simulink model "NEw"  (R2023a)
settings: Solver=FixedStepAuto  StartTime=0.0  StopTime=10  FixedStep=0.01  RelTol=1e-3  EnableMultiTasking=on
libraries: arduinolib x5, arduinosensorlib x1, SignalEditorBlockLib x1
settings Model: ExtModeTrigDuration=2  Creator=abdal  LastModifiedBy=abdal
settings OptimizationCC: EnhancedBackFolding=on  PassReuseOutputArgsAs=Individual arguments  ZeroExternalMemoryAtStartup=off  ZeroInternalMemoryAtStartup=off  MaxStackSize=64  OptimizeBlockOrder=speed  DifferentSizesBufferReuse=on  OptimizationCustomize=off  EfficientTunableParamExpr=on
settings DebuggingCC: ParameterPrecisionLossMsg=none  ParameterTunabilityLossMsg=error
settings HardwareCC: ProdBitPerInt=16  ProdBitPerPointer=16  ProdBitPerSizeT=16  ProdBitPerPtrDiffT=16  ProdLargestAtomicFloat=None  ProdWordSize=8  ProdLongLongMode=on  ProdHWDeviceType=Atmel->AVR
settings SFSimCC: MATLABDynamicMemAlloc=off
settings RTWCC: Description=Embedded Coder  SystemTargetFile=ert.tlc  HardwareBoard=Arduino Uno  TemplateMakefile=ert_default_tmf  Toolchain=Arduino AVR  BuildConfiguration=Faster Runs
settings CodeAppCC: ForceParamTrailComments=on  IgnoreCustomStorageClasses=off  OperatorAnnotations=on  SimulinkDataObjDesc=on  SFDataObjDesc=on  InsertBlockDesc=on
settings ERTTargetCC: SupportContinuousTime=on  SupportVariableSizeSignals=on  ExtModeTransport=3  ExtModeStaticAlloc=on  ExtModeAutomaticAllocSize=off  ExtModeStaticAllocSize=250  ExtModeMexFile=ext_xcp  ExtModeIntrfLevel=Level2 - Open

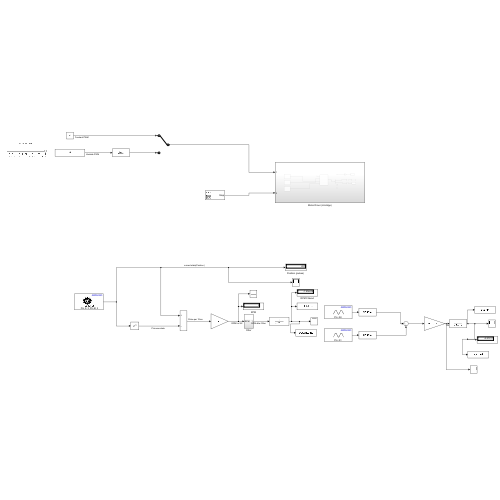
[thumbnail: Simulink's stored preview of the top-level diagram]
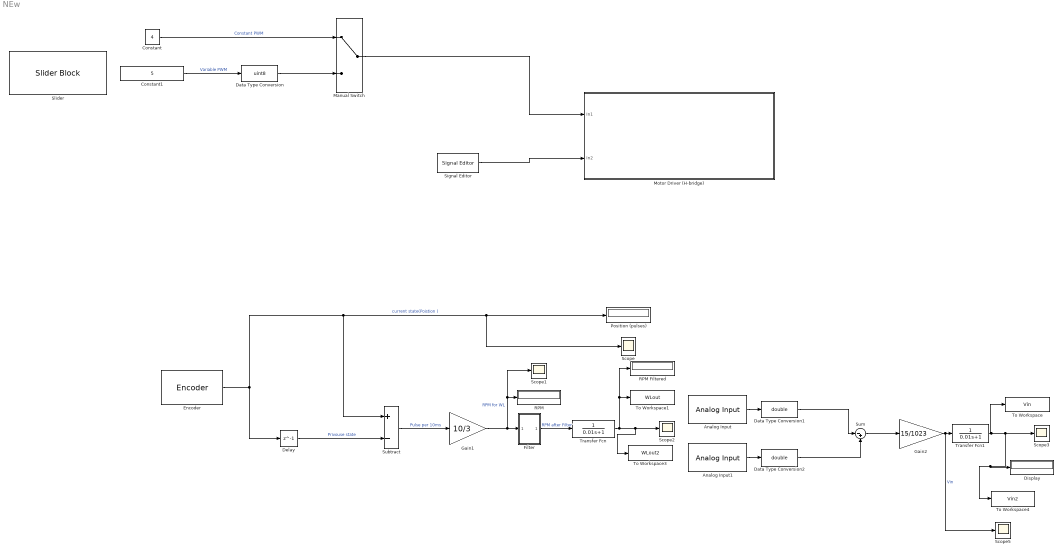
== system NEw ==
  Analog Input : arduinolib/Analog Input  pinNumber=0  ReadResultsOnly=off  ConversionTriggerSource=Software  ExternalTriggerType=uint32( 0 )  OutputDataType=uint16  EnableConversionCompleteNotify=off  EnableOuputStatus=off  SampleTime=-1  blockPlatform=arduino
  Analog Input1 : arduinolib/Analog Input  pinNumber=1  ReadResultsOnly=off  ConversionTriggerSource=Software  ExternalTriggerType=uint32( 0 )  OutputDataType=uint16  EnableConversionCompleteNotify=off  EnableOuputStatus=off  SampleTime=-1  blockPlatform=arduino
  Constant : Constant  Value=4
  Constant1 : Constant  Value=5
  Data Type Conversion : DataTypeConversion  OutMin=0  OutMax=255  OutDataTypeStr=uint8  RndMeth=Simplest  SaturateOnIntegerOverflow=off
  Data Type Conversion1 : DataTypeConversion  OutDataTypeStr=double  SaturateOnIntegerOverflow=off  RndMeth=Floor
  Data Type Conversion2 : DataTypeConversion  OutDataTypeStr=double  SaturateOnIntegerOverflow=off  RndMeth=Floor
  Delay : Delay  DelayLength=1
  Display : Display
  Encoder : arduinosensorlib/Encoder  InputA=3  InputB=2  Mode=No reset  SampleTime=-1
  Filter : Subsystem
  Gain1 : Gain  Gain=10/3
  Gain2 : Gain  Gain=15/1023
  Manual Switch : ManualSwitch
  Motor Driver (H-bridge) : Subsystem
  "Position (pulses) " : Display
  RPM : Display
  RPM Filtered : Display
  Scope{,1..3,5} (5 alike) : Scope
  Signal Editor : SignalEditorBlockLib/Signal Editor  FileName=signal.mat  ActiveScenario=step  ActiveSignal=Step  IsBus=off  OutputBusObjectStr=Bus: BusObject  SampleTime=0  Interpolate=off  ZeroCross=off  OutputAfterFinalValue=Setting to zero  Unit=inherit  PreserveSignalName=on  ApplySigPropsToAllScenarios=on
  Slider : SliderBlock  ScaleMax=5
  Subtract : Sum  Inputs=+-
  Sum : Sum  Inputs=|-+
  To Workspace : ToWorkspace  VariableName=Vin  SampleTime=-1
      settings: Save2DSignal=2-D array (concatenate along first dimension)
  To Workspace1 : ToWorkspace  VariableName=WLout  SampleTime=-1
      settings: Save2DSignal=2-D array (concatenate along first dimension)
  To Workspace3 : ToWorkspace  VariableName=WLout2  SampleTime=-1
      settings: Save2DSignal=2-D array (concatenate along first dimension)
  To Workspace4 : ToWorkspace  VariableName=Vin2  SampleTime=-1
      settings: Save2DSignal=2-D array (concatenate along first dimension)
  Transfer Fcn : TransferFcn  Denominator=[0.01 1]
  Transfer Fcn1 : TransferFcn  Denominator=[0.01 1]
  wires:
  Encoder/1 -> Delay/1, Subtract/1, Scope/1, "Position (pulses) "/1  "current state(Poistion )"
  Delay/1 -> Subtract/2  "Privouse state"
  Subtract/1 -> Gain1/1  "Pulse per 10ms"
  Gain1/1 -> RPM/1, Scope1/1, Filter/1(RPM)  "RPM for WL"
  Filter/1(Out1) -> Transfer Fcn/1  "RPM after Filter"
  Manual Switch/1 -> Motor Driver (H-bridge)/1(In1)
  Constant/1 -> Manual Switch/1  "Constant PWM"
  Constant1/1 -> Data Type Conversion/1  "Variable PWM"
  Data Type Conversion/1 -> Manual Switch/2
  Signal Editor/1 -> Motor Driver (H-bridge)/2(In2)
  Analog Input/1 -> Data Type Conversion1/1
  Analog Input1/1 -> Data Type Conversion2/1
  Sum/1 -> Gain2/1
  Gain2/1 -> Scope5/1, Transfer Fcn1/1  "Vin"
  Data Type Conversion1/1 -> Sum/1
  Data Type Conversion2/1 -> Sum/2
  Transfer Fcn/1 -> To Workspace3/1, Scope2/1, RPM Filtered/1, To Workspace1/1
  Transfer Fcn1/1 -> To Workspace4/1, Display/1, Scope3/1, To Workspace/1

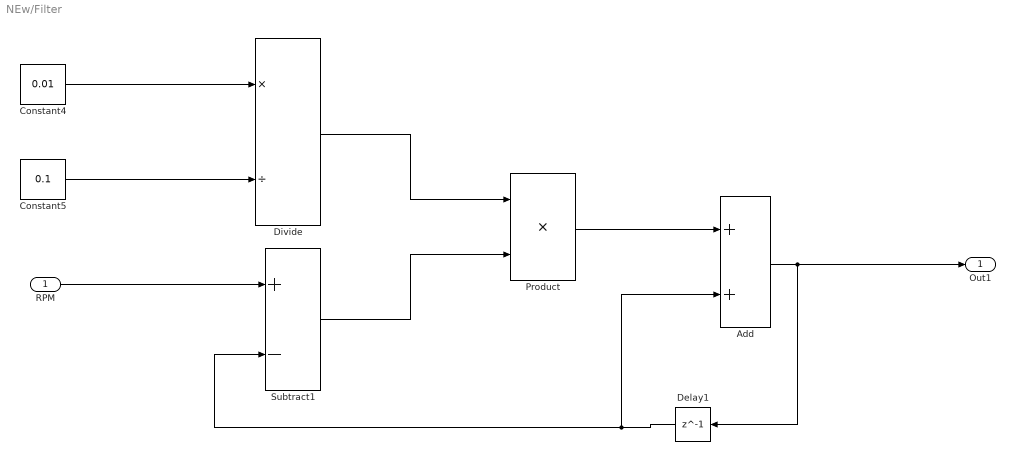
== system NEw/Filter ==
  RPM : Inport
  Add : Sum
  Constant4 : Constant  Value=0.01
  Constant5 : Constant  Value=0.1
  Delay1 : Delay  DelayLength=1
  Divide : Product  Inputs=*/
  Product : Product
  Subtract1 : Sum  Inputs=+-
  Out1 : Outport
  wires:
  RPM/1 -> Subtract1/1
  Subtract1/1 -> Product/2
  Constant4/1 -> Divide/1
  Add/1 -> Out1/1, Delay1/1
  Product/1 -> Add/1
  Divide/1 -> Product/1
  Delay1/1 -> Add/2, Subtract1/2
  Constant5/1 -> Divide/2

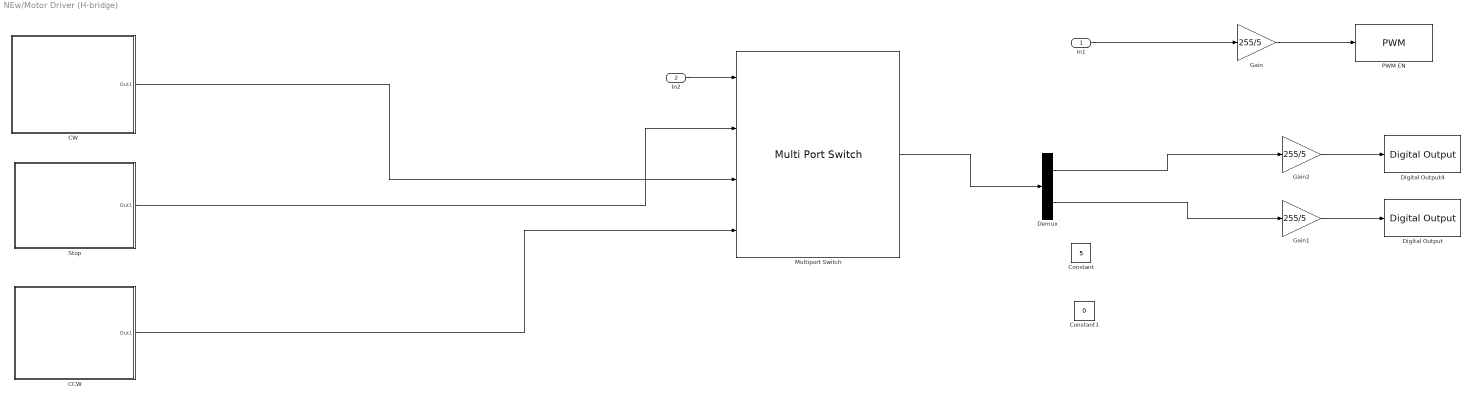
== system NEw/Motor Driver (H-bridge) ==
  In1 : Inport
  In2 : Inport  Port=2
  CCW : Subsystem
  CW : Subsystem
  Constant : Constant  Value=5
  Constant1 : Constant  Value=0
  Demux : Demux  Outputs=2
  Digital Output : arduinolib/Digital Output  pinNumber=9  Direction=output  blockPlatform=arduino
  Digital Output4 : arduinolib/Digital Output  pinNumber=7  Direction=output  blockPlatform=arduino
  Gain : Gain  Gain=255/5
  Gain1 : Gain  Gain=255/5
  Gain2 : Gain  Gain=255/5
  Multiport Switch : MultiPortSwitch  DataPortOrder=Zero-based contiguous  zeroidx=on  SaturateOnIntegerOverflow=off  InputSameDT=off
  PWM EN : arduinolib/PWM  pinNumber=6  frequencyType=Default  desiredFrequency=490.2  achievableFrequency=490.2
  Stop : Subsystem
  wires:
  In1/1 -> Gain/1
  Gain/1 -> PWM EN/1
  Gain1/1 -> Digital Output/1
  Gain2/1 -> Digital Output4/1
  Multiport Switch/1 -> Demux/1
  Demux/1 -> Gain2/1
  Demux/2 -> Gain1/1
  CCW/1(Out1) -> Multiport Switch/4
  CW/1(Out1) -> Multiport Switch/3
  Stop/1(Out1) -> Multiport Switch/2
  In2/1 -> Multiport Switch/1

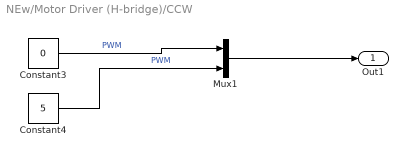
== system NEw/Motor Driver (H-bridge)/CCW ==
  Constant3 : Constant  Value=0
  Constant4 : Constant  Value=5
  Mux1 : Mux  Inputs=2
  Out1 : Outport
  wires:
  Constant4/1 -> Mux1/2  "PWM"
  Mux1/1 -> Out1/1
  Constant3/1 -> Mux1/1  "PWM"

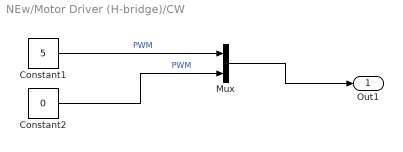
== system NEw/Motor Driver (H-bridge)/CW ==
  Constant1 : Constant  Value=5
  Constant2 : Constant  Value=0
  Mux : Mux  Inputs=2
  Out1 : Outport
  wires:
  Mux/1 -> Out1/1
  Constant1/1 -> Mux/1  "PWM"
  Constant2/1 -> Mux/2  "PWM"

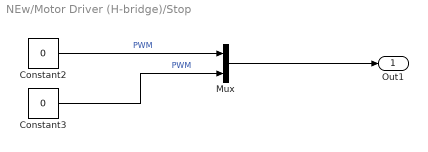
== system NEw/Motor Driver (H-bridge)/Stop ==
  Constant2 : Constant  Value=0
  Constant3 : Constant  Value=0
  Mux : Mux  Inputs=2
  Out1 : Outport
  wires:
  Mux/1 -> Out1/1
  Constant3/1 -> Mux/2  "PWM"
  Constant2/1 -> Mux/1  "PWM"
